simulink model "slave_task"  (Simulink 7.1)
libraries: mathlib x12
settings Model: Creator=jsobota  LastModifiedBy=jsobota  ExtModeTrigMode=oneshot  ExtModeArmWhenConnect=off

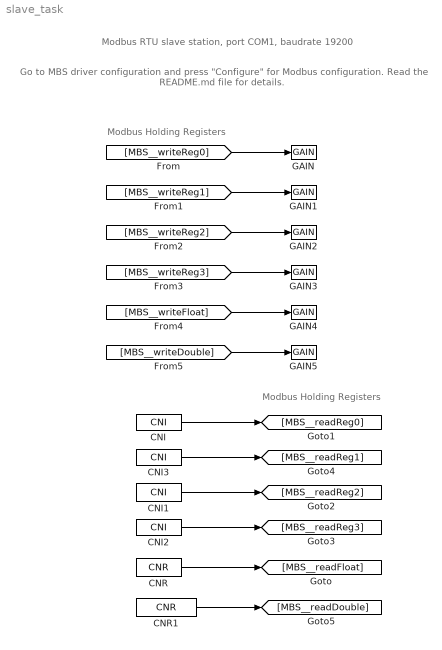
== system slave_task ==
  note: Modbus RTU slave station, port COM1, baudrate 19200
  note: Modbus Holding Registers
  note: Modbus Holding Registers
  note: Go to MBS driver configuration and press "Configure" for Modbus configuration.
      |
      | Read the README.md file for details.
  CNI : mathlib/CNI  icn=91
  CNI1 : mathlib/CNI  icn=65432
  CNI2 : mathlib/CNI  icn=-32132
  CNI3 : mathlib/CNI  icn=-76
  CNR : mathlib/CNR  ycn=-32.76
  CNR1 : mathlib/CNR  ycn=-98765.2
  GAIN{,1..5} (6 alike) : mathlib/GAIN  k=1
  wires:
  CNI/1 -> [MBS__readReg0]
  CNI1/1 -> [MBS__readReg2]
  CNI2/1 -> [MBS__readReg3]
  CNI3/1 -> [MBS__readReg1]
  CNR/1 -> [MBS__readFloat]
  CNR1/1 -> [MBS__readDouble]
  [MBS__writeReg0] -> GAIN/1
  [MBS__writeReg1] -> GAIN1/1
  [MBS__writeReg2] -> GAIN2/1
  [MBS__writeReg3] -> GAIN3/1
  [MBS__writeFloat] -> GAIN4/1
  [MBS__writeDouble] -> GAIN5/1
